simulink model "step4"  (R2021b)
settings: Solver=VariableStepAuto  StartTime=0.0  StopTime=10.0  RelTol=1e-3
settings Model: Creator=just cookie file  LastModifiedBy=just cookie file

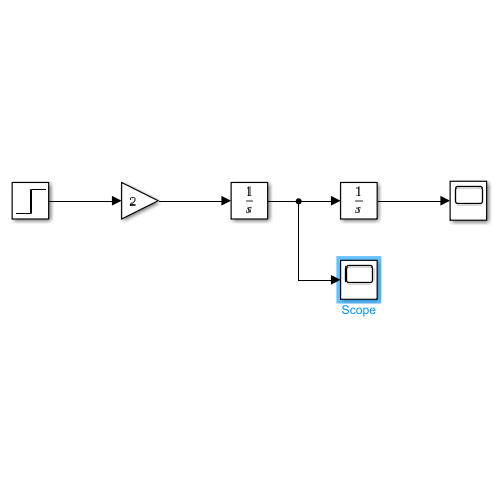
[thumbnail: Simulink's stored preview of the top-level diagram]
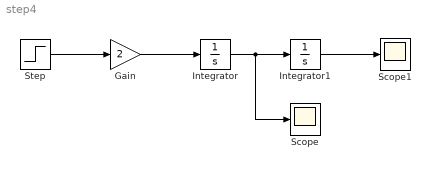
== system step4 ==
  Gain : Gain  Gain=2
  Integrator : Integrator  InitialCondition=1
  Integrator1 : Integrator
  Scope : Scope
  Scope1 : Scope
  Step : Step  SampleTime=0
  wires:
  Step/1 -> Gain/1
  Gain/1 -> Integrator/1
  Integrator/1 -> Scope/1, Integrator1/1
  Integrator1/1 -> Scope1/1
